simulink model "EngineCoolantTemperature"  (R2018a)
settings: Solver=FixedStepDiscrete  StartTime=0.0  StopTime=10.0  RelTol=1e-3
libraries: simulink x5
settings Model: Creator=Sohan  LastModifiedBy=Sohan

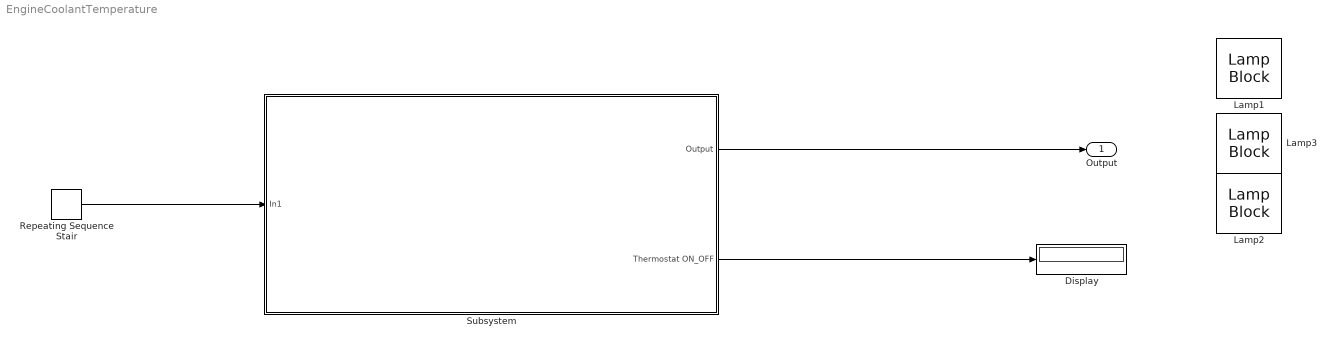
== system EngineCoolantTemperature ==
  Display : Display
  Lamp1 : LampBlock  WebBlockId=19
  Lamp2 : LampBlock  WebBlockId=20
  Lamp3 : LampBlock  WebBlockId=21
  Repeating Sequence Stair : simulink/Sources/Repeating Sequence Stair  OutValues=[20 40 60 80 93 96 99 103 108 109 109 113 50 65 93 98].'  tsamp=-1  OutMin=[]  OutMax=[]  OutDataTypeStr=uint8  OutputDataTypeScalingMode=uint8  OutDataType=fixdt(0,8,1,0.001)  ConRadixGroup=Best Precision: Vector-wise  OutScaling=[]
  Subsystem : Subsystem  TreatAsAtomicUnit=on
  Output : Outport
  wires:
  Repeating Sequence Stair/1 -> Subsystem/1(In1)
  Subsystem/1(Output) -> Output/1
  Subsystem/2(Thermostat ON_OFF) -> Display/1

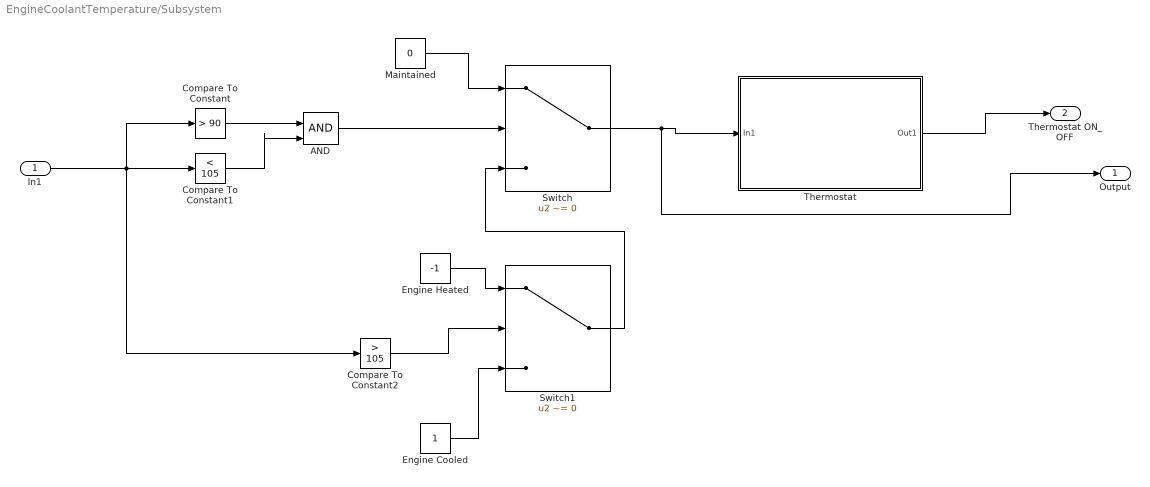
== system EngineCoolantTemperature/Subsystem ==
  In1 : Inport
  AND : Logic  IconShape=distinctive  AllPortsSameDT=off  OutDataTypeStr=boolean
  Compare To Constant : simulink/Logic and Bit Operations/Compare To Constant  relop=>  const=90  OutDataTypeStr=boolean
  Compare To Constant1 : simulink/Logic and Bit Operations/Compare To Constant  relop=<  const=105  OutDataTypeStr=boolean
  Compare To Constant2 : simulink/Logic and Bit Operations/Compare To Constant  relop=>  const=105  OutDataTypeStr=boolean
  Engine Cooled : Constant
  Engine Heated : Constant  Value=-1
  Maintained : Constant  Value=0
  Switch : Switch  Criteria=u2 ~= 0
  Switch1 : Switch  Criteria=u2 ~= 0
  Thermostat : Subsystem
  Output : Outport
  Thermostat ON_OFF : Outport  Port=2
  wires:
  Compare To Constant1/1 -> AND/2
  Compare To Constant/1 -> AND/1
  Maintained/1 -> Switch/1
  Engine Cooled/1 -> Switch1/3
  Switch1/1 -> Switch/3
  In1/1 -> Compare To Constant2/1, Compare To Constant/1, Compare To Constant1/1
  AND/1 -> Switch/2
  Engine Heated/1 -> Switch1/1
  Compare To Constant2/1 -> Switch1/2
  Switch/1 -> Output/1, Thermostat/1(In1)
  Thermostat/1(Out1) -> Thermostat ON_OFF/1

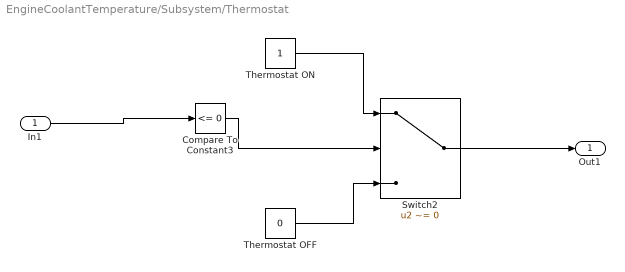
== system EngineCoolantTemperature/Subsystem/Thermostat ==
  In1 : Inport
  Compare To Constant3 : simulink/Logic and Bit Operations/Compare To Constant  relop=<=  const=0  OutDataTypeStr=boolean
  Switch2 : Switch  Criteria=u2 ~= 0  Threshold=-1
  Thermostat OFF : Constant  Value=0
  Thermostat ON : Constant
  Out1 : Outport
  wires:
  Compare To Constant3/1 -> Switch2/2
  In1/1 -> Compare To Constant3/1
  Thermostat ON/1 -> Switch2/1
  Thermostat OFF/1 -> Switch2/3
  Switch2/1 -> Out1/1
